simulink model "optimum_filter_simulink2"  (R2017a)
settings: Solver=VariableStepDiscrete  StartTime=0.0  StopTime=inf  RelTol=1e-3
values from neighbouring files (symbols this model uses):
  gammag = 0.3*pi/180    (= 0.00523598775598)    [optimum_filter3.m]
  h_u = [fliplr(h_ucf(2:end)) 2*h_ucf(1) h_ucf(2:end)]    [optimum_filter3.m]
  K = length(h_ucf)-1    [optimum_filter3.m]
  P = 1    [optimum_filter3.m]
undefined symbols (not defined in the file or in its folder): jsin, magnitude
libraries: dspstat3 x3, dspmathops x3, commchan3 x1, dspsrcs4 x1, dspsigops x1
settings Model: Creator=Shu  LastModifiedBy=mdval
settings DataIOCC: LimitDataPoints=on  SaveOutput=off  SaveTime=off
settings OptimizationCC: BooleanDataType=off  DefaultParameterBehavior=Inlined  LocalBlockOutputs=off  LifeSpan=inf
settings DebuggingCC: AlgebraicLoopMsg=error  SingleTaskRateTransMsg=error  AllowSymbolicDim=off  SFUnexpectedBacktrackingDiag=warning  SFNoUnconditionalDefaultTransitionDiag=warning  SFExecutionAtInitializationDiag=none
settings GRTTargetCC: TargetLangStandard=C89/C90 (ANSI)  GeneratePreprocessorConditionals=Disable all
settings ConfigComp: CovMetricSettings=dw  CovHtmlReporting=on  CovSaveCumulativeToWorkspaceVar=on  CovSaveSingleToWorkspaceVar=on  CovExternalEMLEnable=off  CovSFcnEnable=off

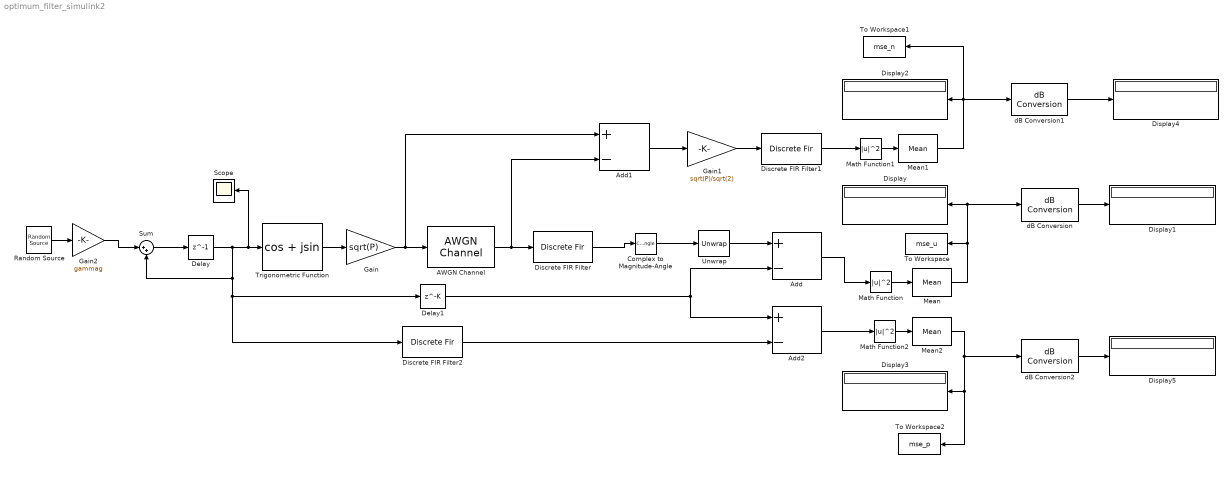
== system optimum_filter_simulink2 ==
  AWGN Channel : commchan3/AWGN Channel  InputProcessing=Columns as channels (frame based)  seed=67  noiseMode="Signal to noise ratio  (SNR)"  EbNodB=10  EsNodB=10  SNRdB=SNRdB  bitsPerSym=1  Ps=1  Tsym=1  variance=1
  Add : Sum  Inputs=+-
  Add1 : Sum  Inputs=+-
  Add2 : Sum  Inputs=+-
  Complex to Magnitude-Angle : ComplexToMagnitudeAngle  Output=Angle
  Delay : Delay  DelayLength=1  InitialCondition=0
  Delay1 : Delay  DelayLength=K  InitialCondition=0
  Discrete FIR Filter : DiscreteFir  Coefficients=h_u  InputProcessing=Columns as channels (frame based)
  Discrete FIR Filter1 : DiscreteFir  Coefficients=h_u  InputProcessing=Columns as channels (frame based)
  Discrete FIR Filter2 : DiscreteFir  Coefficients=h_u  InputProcessing=Columns as channels (frame based)
  Display{,1..5} (6 alike) : Display
  Gain : Gain  Gain=sqrt(P)
  Gain1 : Gain  Gain=sqrt(P)/sqrt(2)
  Gain2 : Gain  Gain=gammag
  Math Function : Math  Operator=magnitude^2  SaturateOnIntegerOverflow=on
  Math Function1 : Math  Operator=magnitude^2  SaturateOnIntegerOverflow=on
  Math Function2 : Math  Operator=magnitude^2  SaturateOnIntegerOverflow=on
  Mean : dspstat3/Mean  run=on  reset_popup=None  InputProcessing=Columns as channels (frame based)  directionMode=Each column  dimension=1  roiEnable=off  roiType=Rectangles  roiPortion=Entire ROI  roiOutput=Individual statistics for each ROI  roiFlag=off  outputDataTypeStr=Inherit: Same as accumulator  outputLastDataTypeStr=Inherit: Same as accumulator  outputMin=[]  outputMax=[]  roundingMode=Floor  overflowMode=off
  Mean1 : dspstat3/Mean  run=on  reset_popup=None  InputProcessing=Columns as channels (frame based)  directionMode=Each column  dimension=1  roiEnable=off  roiType=Rectangles  roiPortion=Entire ROI  roiOutput=Individual statistics for each ROI  roiFlag=off  outputDataTypeStr=Inherit: Same as accumulator  outputLastDataTypeStr=Inherit: Same as accumulator  outputMin=[]  outputMax=[]  roundingMode=Floor  overflowMode=off
  Mean2 : dspstat3/Mean  run=on  reset_popup=None  InputProcessing=Columns as channels (frame based)  directionMode=Each column  dimension=1  roiEnable=off  roiType=Rectangles  roiPortion=Entire ROI  roiOutput=Individual statistics for each ROI  roiFlag=off  outputDataTypeStr=Inherit: Same as accumulator  outputLastDataTypeStr=Inherit: Same as accumulator  outputMin=[]  outputMax=[]  roundingMode=Floor  overflowMode=off
  Random Source : dspsrcs4/Random Source  SrcType=Gaussian  NormMethod=Ziggurat  CltLength=12  MinVal=0  MaxVal=1  MeanVal=0  VarVal=1  RepMode=Not repeatable  rawSeed=1  IsInherit=off  SampMode=Discrete  SampTime=1  SampFrame=1  DataType=Double  OutComplex=Real  OutputFrames=off
  Scope : Scope
  Sum : Sum  Inputs=|++
  To Workspace : ToWorkspace  VariableName=mse_u  SampleTime=-1
      settings: MaxDataPoints=1
  To Workspace1 : ToWorkspace  VariableName=mse_n  SampleTime=-1
      settings: MaxDataPoints=1
  To Workspace2 : ToWorkspace  VariableName=mse_p  SampleTime=-1
      settings: MaxDataPoints=1
  Trigonometric Function : Trigonometry  Operator=cos + jsin
  Unwrap : dspsigops/Unwrap  tol=pi  InputProcessing=Columns as channels (frame based)  running=off
  dB Conversion : dspmathops/dB Conversion  dBtype=dB  intype=Power  R=1  fuzz=on
      settings: SourceProductName=DSP System Toolbox
  dB Conversion1 : dspmathops/dB Conversion  dBtype=dB  intype=Power  R=1  fuzz=on
      settings: SourceProductName=DSP System Toolbox
  dB Conversion2 : dspmathops/dB Conversion  dBtype=dB  intype=Power  R=1  fuzz=on
      settings: SourceProductName=DSP System Toolbox
  wires:
  Trigonometric Function/1 -> Gain/1
  Gain/1 -> Add1/1, AWGN Channel/1
  AWGN Channel/1 -> Add1/2, Discrete FIR Filter/1
  Random Source/1 -> Gain2/1
  Gain2/1 -> Sum/1
  Sum/1 -> Delay/1
  Delay/1 -> Discrete FIR Filter2/1, Delay1/1, Sum/2, Scope/1, Trigonometric Function/1
  Complex to Magnitude-Angle/1 -> Unwrap/1
  Discrete FIR Filter/1 -> Complex to Magnitude-Angle/1
  Unwrap/1 -> Add/1
  Add/1 -> Math Function/1
  Math Function/1 -> Mean/1
  Mean/1 -> dB Conversion/1, Display/1, To Workspace/1
  dB Conversion/1 -> Display1/1
  Add1/1 -> Gain1/1
  Discrete FIR Filter1/1 -> Math Function1/1
  Gain1/1 -> Discrete FIR Filter1/1
  Math Function1/1 -> Mean1/1
  Mean1/1 -> Display2/1, To Workspace1/1, dB Conversion1/1
  Discrete FIR Filter2/1 -> Add2/2
  Delay1/1 -> Add2/1, Add/2
  Add2/1 -> Math Function2/1
  Math Function2/1 -> Mean2/1
  dB Conversion1/1 -> Display4/1
  Mean2/1 -> To Workspace2/1, Display3/1, dB Conversion2/1
  dB Conversion2/1 -> Display5/1
